simulink model "hybrid_lht_accumulator_backup"  (R2019b)
settings: Solver=FixedStepDiscrete  StartTime=0.0  StopTime=inf  FixedStep=1/bt.frequency  RelTol=1e-3
InitFcn:
  | ht_hybrid_setup;
StopFcn:
  | ht_hybrid_compare;
undefined symbols (not defined in the file or in its folder): bt, height, Ntheta, nTheta, width
libraries: hdlsllib x52, simulink x24, visionhdlutilities x2, dspsrcs4 x1, visionhdlio x1, lib_hybrid_ht_kernel x1, visionsources x1
(part 3 of 5)

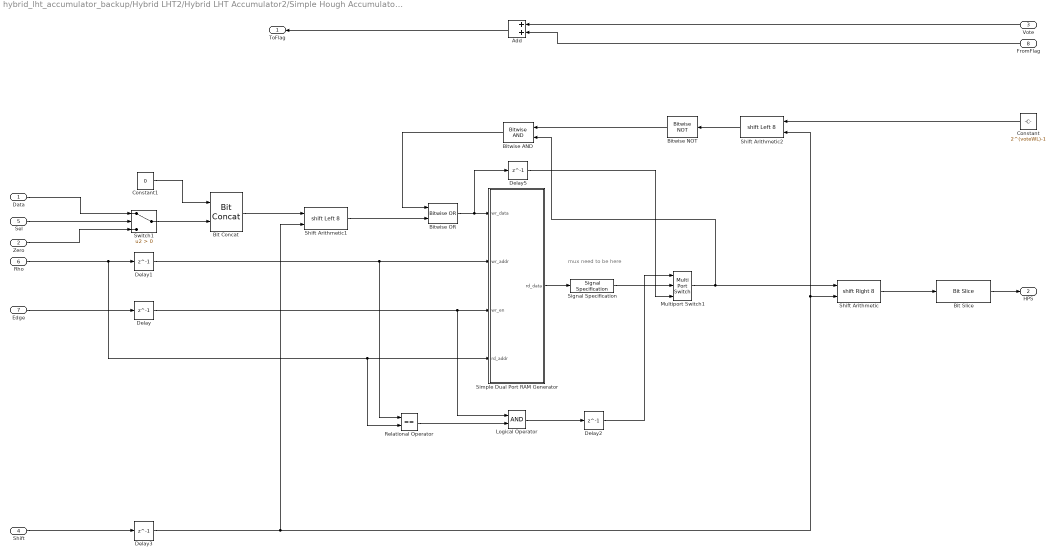
== system hybrid_lht_accumulator_backup/Hybrid LHT2/Hybrid LHT Accumulator2/Simple Hough Accumulator/Hough Accumulator ==
  note: mux need to be here
  Data : Inport
  Zero : Inport  Port=2
  Vote : Inport  Port=3
  Shift : Inport  Port=4
  Sel : Inport  Port=5
  Rho : Inport  Port=6
  Edge : Inport  Port=7
  FromFlag : Inport  Port=8
  Add : Sum  OutDataTypeStr=fixdt(0,voteWL,0)
  Bit Concat : hdlsllib/Logic and Bit Operations/Bit Concat  numInputs=2
      settings: SourceProductName=HDL Coder  SourceProductBaseCode=HD
  Bit Slice : hdlsllib/Logic and Bit Operations/Bit Slice  lidx=voteWL-1  ridx=0
  Bitwise AND : simulink/Logic and Bit Operations/Bitwise Operator  logicop=AND  UseBitMask=off  NumInputPorts=2  BitMask=bin2dec('11011001')  BitMaskRealWorld=Stored Integer
  Bitwise NOT : simulink/Logic and Bit Operations/Bitwise Operator  logicop=NOT  UseBitMask=off  BitMask=bin2dec('11011001')  BitMaskRealWorld=Stored Integer
  Bitwise OR : simulink/Logic and Bit Operations/Bitwise Operator  logicop=OR  UseBitMask=off  NumInputPorts=2  BitMask=bin2dec('11011001')  BitMaskRealWorld=Stored Integer
  Constant : Constant  Value=2^(voteWL)-1  OutDataTypeStr=fixdt(0, 36, 0)  SampleTime=-1
  Constant1 : Constant  Value=0  OutDataTypeStr=fixdt(0, 36-voteWL, 0)  SampleTime=-1
  Delay{,1..3,5} (5 alike) : Delay  DelayLength=1
  Logical Operator : Logic  AllPortsSameDT=off  OutDataTypeStr=boolean
  Multiport Switch1 : MultiPortSwitch  DataPortOrder=Zero-based contiguous  Inputs=2  zeroidx=on
  Relational Operator : RelationalOperator  Operator===  OutDataTypeStr=boolean  RndMeth=Simplest
  Shift Arithmetic : ArithShift  BitShiftNumberSource=Input port  BitShiftNumber=8  BitShiftDirection=Right  DiagnosticForOORShift=Error
      settings: InputPortMap=u0,p1
  Shift Arithmetic1 : ArithShift  BitShiftNumberSource=Input port  BitShiftNumber=8  BitShiftDirection=Left  DiagnosticForOORShift=Error
      settings: InputPortMap=u0,p1
  Shift Arithmetic2 : ArithShift  BitShiftNumberSource=Input port  BitShiftNumber=8  BitShiftDirection=Left  DiagnosticForOORShift=Error
      settings: InputPortMap=u0,p1
  Signal Specification : SignalSpecification  OutDataTypeStr=fixdt(0, 36, 0)
  Simple Dual Port RAM Generator : Subsystem  mask{b=36, d=Nrho}
      mask prompts: b "Data width:"; d "Depth:"
      mask init: same as hybrid_lht_accumulator_backup/Hybrid LHT/Hybrid LHT Accumulator/Simple Hough Accumulator/Hough Accumulator/Simple Dual Port RAM Generator
  Switch1 : Switch  Criteria=u2 > Threshold
  ToFlag : Outport  VectorParamsAs1DForOutWhenUnconnected=off
  HPS : Outport  Port=2  VectorParamsAs1DForOutWhenUnconnected=off
  wires:
  Delay2/1 -> Multiport Switch1/1
  Delay1/1 -> Relational Operator/1, Simple Dual Port RAM Generator/2(wr_addr)
  Relational Operator/1 -> Logical Operator/2
  Add/1 -> ToFlag/1
  Edge/1 -> Delay/1
  FromFlag/1 -> Add/2
  Sel/1 -> Switch1/2
  Vote/1 -> Add/1
  Data/1 -> Switch1/1
  Zero/1 -> Switch1/3
  Shift Arithmetic/1 -> Bit Slice/1
  Simple Dual Port RAM Generator/1(rd_data) -> Signal Specification/1
  Switch1/1 -> Bit Concat/2
  Logical Operator/1 -> Delay2/1
  Shift/1 -> Delay3/1
  Delay3/1 -> Shift Arithmetic2/2, Shift Arithmetic/2, Shift Arithmetic1/2
  Shift Arithmetic1/1 -> Bitwise OR/2
  Bitwise AND/1 -> Bitwise OR/1
  Bit Concat/1 -> Shift Arithmetic1/1
  Constant1/1 -> Bit Concat/1
  Shift Arithmetic2/1 -> Bitwise NOT/1
  Constant/1 -> Shift Arithmetic2/1
  Bitwise NOT/1 -> Bitwise AND/1
  Delay/1 -> Logical Operator/1, Simple Dual Port RAM Generator/3(wr_en)
  Bit Slice/1 -> HPS/1
  Signal Specification/1 -> Multiport Switch1/2
  Multiport Switch1/1 -> Bitwise AND/2, Shift Arithmetic/1
  Bitwise OR/1 -> Delay5/1, Simple Dual Port RAM Generator/1(wr_data)
  Delay5/1 -> Multiport Switch1/3
  Rho/1 -> Delay1/1, Relational Operator/2, Simple Dual Port RAM Generator/4(rd_addr)

== system hybrid_lht_accumulator_backup/Hybrid LHT2/Hybrid LHT Accumulator2/Simple Hough Accumulator/Keep Flag ==
  "FlagIn " : Inport
  "VoteIn " : Inport  Port=2
  Keep Flag : Subsystem  VariantControl=Backprojection
  Passthrough : Subsystem  VariantControl=Passthrough
  " VoteFlagOut" : Outport  VectorParamsAs1DForOutWhenUnconnected=off

== system hybrid_lht_accumulator_backup/Hybrid LHT2/Hybrid LHT Accumulator2/Simple Hough Accumulator/Separate Bits ==
  "VoteFlagIn " : Inport
  Passthrough : Subsystem  VariantControl=Passthrough
  Separate Bits : Subsystem  VariantControl=Backprojection
  " FlagOut" : Outport  VectorParamsAs1DForOutWhenUnconnected=off
  " VoteOut" : Outport  Port=2  VectorParamsAs1DForOutWhenUnconnected=off

== system hybrid_lht_accumulator_backup/Hybrid LHT2/Hybrid LHT Kernel/Extract Active Votes/GetShift ==
  Theta : Inport
  Add : Sum  Inputs=+  OutDataTypeStr=fixdt(0, ceil(log2(L+1)), 0)
  Constant : Constant  Value=U  VectorParams1D=off  OutDataTypeStr=fixdt(0,ceil(log2(max(U)+1)),0)  SampleTime=-1
  Relational Operator : RelationalOperator  OutDataTypeStr=boolean  RndMeth=Nearest
  Shift : Outport  VectorParamsAs1DForOutWhenUnconnected=off
  wires:
  Relational Operator/1 -> Add/1
  Add/1 -> Shift/1
  Theta/1 -> Relational Operator/1
  Constant/1 -> Relational Operator/2

== system hybrid_lht_accumulator_backup/Hybrid LHT2/Hybrid LHT Kernel/Gradient Kernel System/Get Index and Fix Limits ==
  Theta : Inport
  Data Type Conversion : DataTypeConversion  OutDataTypeStr=uint16
  Extract Active Votes : Subsystem
  Gain : Gain  Gain=fi(voteWL, 0, 6, 0)  ParamDataTypeStr=fixdt(0,6,0)  OutDataTypeStr=fixdt(0, 6, 0)
  GetShift1 : Subsystem
  Index : Outport  VectorParamsAs1DForOutWhenUnconnected=off
  Shift : Outport  Port=2  VectorParamsAs1DForOutWhenUnconnected=off
  wires:
  Gain/1 -> Shift/1
  Extract Active Votes/1(Index) -> GetShift1/1(Theta), Data Type Conversion/1
  Theta/1 -> Extract Active Votes/1(Theta)
  Data Type Conversion/1 -> Index/1
  GetShift1/1(Shift) -> Gain/1

== system hybrid_lht_accumulator_backup/Hybrid LHT2/Hybrid LHT Kernel/Gradient Kernel System/Hough Kernel ==
  Edge : Inport
  X : Inport  Port=2
  Y : Inport  Port=3
  Index : Inport  Port=4
  Add1 : Sum  OutDataTypeStr=fixdt(0, ceil(log2(2*maxRho)), 0)  RndMeth=Round
  Constant : Constant  Value=maxRho  OutDataTypeStr=fixdt(0, ceil(log2(maxRho + 1)), 0);  SampleTime=-1
  Data Type Conversion : DataTypeConversion  OutDataTypeStr=uint16
  Hough Kernel : Subsystem
  vEdge : Outport  VectorParamsAs1DForOutWhenUnconnected=off
  Rho : Outport  Port=2  VectorParamsAs1DForOutWhenUnconnected=off
  wires:
  Edge/1 -> vEdge/1
  Hough Kernel/1(Rho) -> Add1/1
  Data Type Conversion/1 -> Hough Kernel/3(Index)
  Y/1 -> Hough Kernel/2(Y)
  X/1 -> Hough Kernel/1(X)
  Index/1 -> Data Type Conversion/1
  Add1/1 -> Rho/1
  Constant/1 -> Add1/2

== system hybrid_lht_accumulator_backup/Hybrid LHT2/Hybrid LHT Kernel1/Gradient Kernel System/Extract Active Votes ==
  note: Check the indices to ensure they are in the correct limits
  Theta : Inport
  Add : Sum
  Add1 : Sum  Inputs=+-
  Add2 : Sum  Inputs=+-
  Add3 : Sum
  Add4 : Sum  Inputs=+-  OutDataTypeStr=uint16
  Constant : Constant  Value=[-lambda:1:lambda-subflag]  VectorParams1D=off  OutDataTypeStr=fixdt(1,ceil(log2(lambda+1))+1, 0)  SampleTime=-1
  Data Type Conversion : DataTypeConversion  OutDataTypeStr=fixdt(0, ceil(log2(nTheta+1)), 0)
  Data Type Conversion1 : DataTypeConversion  OutDataTypeStr=uint16
  Gain1 : Gain  Gain=nTheta/L  ParamDataTypeStr=fixdt(0, ceil(log2(nTheta+1)), 0)  OutDataTypeStr=fixdt(0, ceil(log2(nTheta+1)), 0)
  GetShift : Subsystem
  High : Constant  Value=nTheta/L-1  OutDataTypeStr=fixdt(0,ceil(log2(nTheta)),0)  SampleTime=-1
  High1 : Constant  Value=nTheta/L-1  OutDataTypeStr=fixdt(0,ceil(log2(nTheta)),0)  SampleTime=-1
  Low : Constant  Value=0  OutDataTypeStr=fixdt(0,1,0)  SampleTime=-1
  Multiport Switch2 : MultiPortSwitch  DataPortOrder=Zero-based contiguous  Inputs=2  zeroidx=on
  Multiport Switch3 : MultiPortSwitch  DataPortOrder=Zero-based contiguous  Inputs=2  zeroidx=on
  Relational : RelationalOperator  Operator=<  OutDataTypeStr=boolean  RndMeth=Nearest
  Relational1 : RelationalOperator  Operator=>  OutDataTypeStr=boolean  RndMeth=Nearest
  Selector4 : Selector  NumberOfDimensions=2  IndexMode=Zero-based  InputPortWidth=3  IndexOptions=Index vector (dialog),Index vector (dialog)  Indices=0,[nTheta/floor(36/ceil(log2(2*maxRho)))-1:-1:0]  OutputSizes=1,1
  nTheta : Constant  Value=nTheta/L  OutDataTypeStr=fixdt(0,ceil(log2(nTheta+1)),0)  SampleTime=-1
  Index : Outport  VectorParamsAs1DForOutWhenUnconnected=off
  wires:
  Data Type Conversion1/1 -> Add4/2
  Data Type Conversion/1 -> Data Type Conversion1/1
  Add4/1 -> Selector4/1
  High1/1 -> Add4/1
  Add2/1 -> Add/1
  Add/1 -> Multiport Switch2/2, Relational/1, Add3/1
  Theta/1 -> GetShift/1(Theta), Add2/1
  nTheta/1 -> Add1/2, Add3/2
  Multiport Switch2/1 -> Multiport Switch3/2, Relational1/1, Add1/1
  Low/1 -> Relational/2
  Add3/1 -> Multiport Switch2/3
  Relational1/1 -> Multiport Switch3/1
  High/1 -> Relational1/2
  Multiport Switch3/1 -> Data Type Conversion/1
  Relational/1 -> Multiport Switch2/1
  Add1/1 -> Multiport Switch3/3
  Constant/1 -> Add/2
  Selector4/1 -> Index/1
  GetShift/1(Shift) -> Gain1/1
  Gain1/1 -> Add2/2

== system hybrid_lht_accumulator_backup/Hybrid LHT2/Hybrid LHT Kernel1/Gradient Kernel System/Get Index and Fix Limits ==
  note: Get the number of bits to shift for write to memory
  Theta : Inport
  Extract Active Votes : Subsystem
  Gain : Gain  Gain=fi(voteWL, 0, 6, 0)  ParamDataTypeStr=fixdt(0,6,0)  OutDataTypeStr=fixdt(0, 6, 0)
  GetShift1 : Subsystem
  Selector1 : Selector  NumberOfDimensions=2  IndexMode=Zero-based  InputPortWidth=3  IndexOptions=Index vector (dialog),Index vector (dialog)  Indices=0,0  OutputSizes=1,1
  Terminator1 : Terminator
  Index : Outport  VectorParamsAs1DForOutWhenUnconnected=off
  Shift : Outport  Port=2  VectorParamsAs1DForOutWhenUnconnected=off
  wires:
  Extract Active Votes/1(Index) -> GetShift1/1(Theta), Index/1, Selector1/1
  Theta/1 -> Extract Active Votes/1(Theta)
  GetShift1/1(Shift) -> Gain/1
  Gain/1 -> Shift/1
  Selector1/1 -> Terminator1/1

== system hybrid_lht_accumulator_backup/Hybrid LHT2/Hybrid LHT Kernel1/Gradient Kernel System/Hough Kernel ==
  Edge : Inport
  X : Inport  Port=2
  Y : Inport  Port=3
  Index : Inport  Port=4
  Add1 : Sum  OutDataTypeStr=fixdt(0, ceil(log2(2*maxRho)), 0)  RndMeth=Round
  Constant : Constant  Value=maxRho  OutDataTypeStr=fixdt(0, ceil(log2(maxRho + 1)), 0);  SampleTime=-1
  Data Type Conversion : DataTypeConversion  OutDataTypeStr=uint16
  Hough Kernel : Subsystem
  vEdge : Outport  VectorParamsAs1DForOutWhenUnconnected=off
  Rho : Outport  Port=2  VectorParamsAs1DForOutWhenUnconnected=off
  wires:
  Constant/1 -> Add1/2
  Add1/1 -> Rho/1
  Index/1 -> Data Type Conversion/1
  X/1 -> Hough Kernel/1(X)
  Y/1 -> Hough Kernel/2(Y)
  Data Type Conversion/1 -> Hough Kernel/3(Index)
  Hough Kernel/1(Rho) -> Add1/1
  Edge/1 -> vEdge/1

== system hybrid_lht_accumulator_backup/Hybrid LHT2/Hybrid LHT Kernel2/Extract Active Votes/GetShift ==
  Theta : Inport
  Add : Sum  Inputs=+  OutDataTypeStr=fixdt(0, ceil(log2(L+1)), 0)
  Constant : Constant  Value=U  VectorParams1D=off  OutDataTypeStr=fixdt(0,ceil(log2(max(U)+1)),0)  SampleTime=-1
  Relational Operator : RelationalOperator  OutDataTypeStr=boolean  RndMeth=Nearest
  Shift : Outport  VectorParamsAs1DForOutWhenUnconnected=off
  wires:
  Relational Operator/1 -> Add/1
  Add/1 -> Shift/1
  Theta/1 -> Relational Operator/1
  Constant/1 -> Relational Operator/2

== system hybrid_lht_accumulator_backup/Hybrid LHT2/Hybrid LHT Kernel2/Gradient Kernel System/Get Index and Fix Limits ==
  Theta : Inport
  Data Type Conversion : DataTypeConversion  OutDataTypeStr=uint16
  Extract Active Votes : Subsystem
  Gain : Gain  Gain=fi(voteWL, 0, 6, 0)  ParamDataTypeStr=fixdt(0,6,0)  OutDataTypeStr=fixdt(0, 6, 0)
  GetShift1 : Subsystem
  Index : Outport  VectorParamsAs1DForOutWhenUnconnected=off
  Shift : Outport  Port=2  VectorParamsAs1DForOutWhenUnconnected=off
  wires:
  GetShift1/1(Shift) -> Gain/1
  Data Type Conversion/1 -> Index/1
  Theta/1 -> Extract Active Votes/1(Theta)
  Extract Active Votes/1(Index) -> Data Type Conversion/1, GetShift1/1(Theta)
  Gain/1 -> Shift/1

== system hybrid_lht_accumulator_backup/Hybrid LHT2/Hybrid LHT Kernel2/Gradient Kernel System/Hough Kernel ==
  Edge : Inport
  X : Inport  Port=2
  ysin : Inport  Port=3
  Index : Inport  Port=4
  Add1 : Sum  OutDataTypeStr=fixdt(0, ceil(log2(2*maxRho)), 0)  RndMeth=Round
  Constant : Constant  Value=maxRho  OutDataTypeStr=fixdt(0, ceil(log2(maxRho + 1)), 0);  SampleTime=-1
  Data Type Conversion : DataTypeConversion  OutDataTypeStr=uint16
  Hough Kernel : Subsystem
  vEdge : Outport  VectorParamsAs1DForOutWhenUnconnected=off
  Rho : Outport  Port=2  VectorParamsAs1DForOutWhenUnconnected=off
  wires:
  Hough Kernel/1(Rho) -> Add1/1
  Data Type Conversion/1 -> Hough Kernel/3(Index)
  ysin/1 -> Hough Kernel/2(Y)
  X/1 -> Hough Kernel/1(X)
  Index/1 -> Data Type Conversion/1
  Constant/1 -> Add1/2
  Add1/1 -> Rho/1
  Edge/1 -> vEdge/1

== system hybrid_lht_accumulator_backup/Hybrid LHT/Hybrid LHT Accumulator/Simple Hough Accumulator/Flag Generator/Flag Generator ==
  ReadOut : Inport
  Thresh : Inport  Port=2
  ZeroData : Inport  Port=3
  ReadValid : Inport  Port=4
  AND : Logic  IconShape=distinctive  AllPortsSameDT=off  OutDataTypeStr=boolean
  Bit Concat : hdlsllib/Logic and Bit Operations/Bit Concat  numInputs=2
      settings: SourceProductName=HDL Coder  SourceProductBaseCode=HD
  Relational Operator1 : RelationalOperator  OutDataTypeStr=boolean  RndMeth=Simplest
  ZeroDataFlagged : Outport  VectorParamsAs1DForOutWhenUnconnected=off
  wires:
  AND/1 -> Bit Concat/1
  ReadValid/1 -> AND/2
  Relational Operator1/1 -> AND/1
  ZeroData/1 -> Bit Concat/2
  Bit Concat/1 -> ZeroDataFlagged/1
  Thresh/1 -> Relational Operator1/2
  ReadOut/1 -> Relational Operator1/1

== system hybrid_lht_accumulator_backup/Hybrid LHT/Hybrid LHT Accumulator/Simple Hough Accumulator/Flag Generator/Passthrough ==
  ZeroData : Inport
  ZeroDataFlagged : Outport  VectorParamsAs1DForOutWhenUnconnected=off
  wires:
  ZeroData/1 -> ZeroDataFlagged/1

== system hybrid_lht_accumulator_backup/Hybrid LHT/Hybrid LHT Accumulator/Simple Hough Accumulator/Hough Accumulator/Simple Dual Port RAM Generator ==
  wr_data : Inport
  wr_addr : Inport  Port=2
  wr_en : Inport  Port=3
  rd_addr : Inport  Port=4
  rd_address : hdlsllib/Logic and Bit Operations/Bit Slice  lidx=8  ridx=0
      settings: SourceProductName=Simulink  SourceProductBaseCode=SL
  simple_ram_0 : hdlsllib/HDL RAMs/Simple Dual Port RAM  ram_size=9
      settings: SourceProductName=Simulink  SourceProductBaseCode=SL
  wr_address : hdlsllib/Logic and Bit Operations/Bit Slice  lidx=8  ridx=0
      settings: SourceProductName=Simulink  SourceProductBaseCode=SL
  rd_data : Outport
  wires:
  wr_data/1 -> simple_ram_0/1
  wr_addr/1 -> wr_address/1
  wr_address/1 -> simple_ram_0/2
  wr_en/1 -> simple_ram_0/3
  rd_addr/1 -> rd_address/1
  rd_address/1 -> simple_ram_0/4
  simple_ram_0/1 -> rd_data/1

== system hybrid_lht_accumulator_backup/Hybrid LHT/Hybrid LHT Accumulator/Simple Hough Accumulator/Keep Flag/Keep Flag ==
  FlagIn : Inport
  VoteIn : Inport  Port=2
  Bit Concat1 : hdlsllib/Logic and Bit Operations/Bit Concat  numInputs=2
      settings: SourceProductName=HDL Coder  SourceProductBaseCode=HD
  VoteFlagOut : Outport  VectorParamsAs1DForOutWhenUnconnected=off
  wires:
  VoteIn/1 -> Bit Concat1/2
  FlagIn/1 -> Bit Concat1/1
  Bit Concat1/1 -> VoteFlagOut/1

== system hybrid_lht_accumulator_backup/Hybrid LHT/Hybrid LHT Accumulator/Simple Hough Accumulator/Keep Flag/Passthrough ==
  FlagIn : Inport
  VoteIn : Inport  Port=2
  Terminator : Terminator
  VoteFlagOut : Outport  VectorParamsAs1DForOutWhenUnconnected=off
  wires:
  VoteIn/1 -> VoteFlagOut/1
  FlagIn/1 -> Terminator/1

== system hybrid_lht_accumulator_backup/Hybrid LHT/Hybrid LHT Accumulator/Simple Hough Accumulator/Separate Bits/Passthrough ==
  VoteFlagIn : Inport
  Constant : Constant  Value=0  OutDataTypeStr=boolean  SampleTime=-1
  FlagOut : Outport  VectorParamsAs1DForOutWhenUnconnected=off
  VoteOut : Outport  Port=2  VectorParamsAs1DForOutWhenUnconnected=off
  wires:
  VoteFlagIn/1 -> VoteOut/1
  Constant/1 -> FlagOut/1

== system hybrid_lht_accumulator_backup/Hybrid LHT/Hybrid LHT Accumulator/Simple Hough Accumulator/Separate Bits/Separate Bits ==
  VoteFlagIn : Inport
  Bit Slice : hdlsllib/Logic and Bit Operations/Bit Slice  lidx=voteWL-2  ridx=0
  Bit Slice1 : hdlsllib/Logic and Bit Operations/Bit Slice  lidx=voteWL-1  ridx=voteWL-1
  FlagOut : Outport  VectorParamsAs1DForOutWhenUnconnected=off
  VoteOut : Outport  Port=2  VectorParamsAs1DForOutWhenUnconnected=off
  wires:
  VoteFlagIn/1 -> Bit Slice/1, Bit Slice1/1
  Bit Slice/1 -> VoteOut/1
  Bit Slice1/1 -> FlagOut/1
